simulink model "Identificacion_Simulink"  (R2016b)
settings: Solver=VariableStepAuto  StartTime=0.0  StopTime=30  FixedStep=Td  RelTol=1e-3
values from neighbouring files (symbols this model uses):
  Td = 0.1    [Initialization_MPC_SS.m]    (also in Script_identificacionW.m)
settings Model: Creator=asierzubizarreta  LastModifiedBy=asierzubizarreta

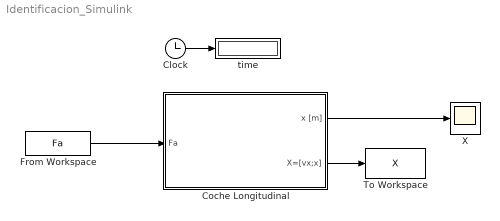
== system Identificacion_Simulink ==
  Clock : Clock
  Coche Longitudinal : Subsystem  SystemSampleTime=Td  mask{m=1000, Br=500, Ka=50000, wlim1=1, wlim2=0.1, Td=0.1}
      mask prompts: m "Mass (m)"; Br "Friction (Br)"; Ka "Motor constant (Ka)"; wlim1 "Max Uncertainty (w_v)"; wlim2 "Max Uncertainty (w_x)"; Td "Discretization Time (Td)"
      mask init:
      | Ac=[-Br/m 0; 1 0];
      | Bc=[Ka/m;0];
      | Cc=eye(2);
      | 
      | %Dscretizaci?n
      | 
      | sc=ss(Ac,Bc,Cc,0);
      | 
      | %% Sistema discretizado:
      | 
      | sd=c2d(sc,Td);
      | A=sd.a;
      | B=sd.b;
      | C=sd.c;
  From Workspace : FromWorkspace  VariableName=Fa  SampleTime=Td
  To Workspace : ToWorkspace  VariableName=X  SaveFormat=Structure With Time  SampleTime=Td
  X : Scope
  time : Display
  wires:
  Clock/1 -> time/1
  Coche Longitudinal/1(x [m]) -> X/1
  Coche Longitudinal/2(X=[vx;x]) -> To Workspace/1
  From Workspace/1 -> Coche Longitudinal/1(Fa)

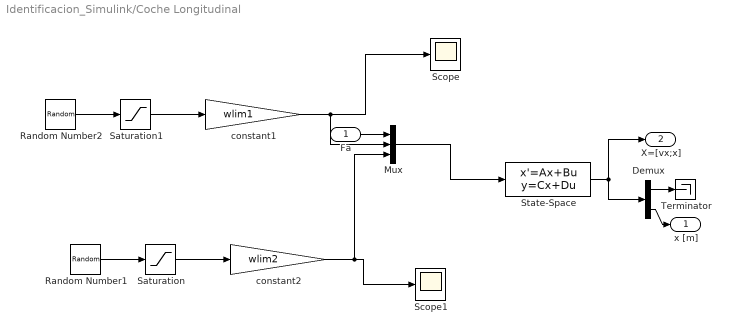
== system Identificacion_Simulink/Coche Longitudinal ==
  Fa : Inport
  Demux : Demux  Outputs=2
  Mux : Mux  Inputs=3
  Random Number1 : RandomNumber  Seed=1  SampleTime=0.1
  Random Number2 : RandomNumber  Seed=0.5  SampleTime=0.1
  Saturation : Saturate  UpperLimit=1  LowerLimit=-1
  Saturation1 : Saturate  UpperLimit=1  LowerLimit=-1
  Scope : Scope
  Scope1 : Scope
  State-Space : StateSpace  A=Ac  B=[Bc eye(2)]  C=eye(2)  D=zeros(2,3)  X0=0
  Terminator : Terminator
  constant1 : Gain  Gain=wlim1
  constant2 : Gain  Gain=wlim2
  x [m] : Outport
  X=[vx;x] : Outport  Port=2
  wires:
  Random Number1/1 -> Saturation/1
  constant1/1 -> Mux/2, Scope/1
  constant2/1 -> Mux/3, Scope1/1
  Demux/1 -> Terminator/1
  Demux/2 -> x [m]/1
  Random Number2/1 -> Saturation1/1
  Saturation1/1 -> constant1/1
  Saturation/1 -> constant2/1
  State-Space/1 -> X=[vx;x]/1, Demux/1
  Fa/1 -> Mux/1
  Mux/1 -> State-Space/1
